simulink model "DroneModelv7"  (R2023b)
settings: Solver=VariableStepAuto  StartTime=10  StopTime=100  FixedStep=0.00001  RelTol=1e-3
undefined symbols (not defined in the file): alpha_vec_Cn0, beta_vec_Cn0, bref, Clbeta, Clda, Cm0, Cmda, Cmde, Cn0, Cnda, CX0, CXda, CXde, CYbeta, CYda, CZ0, CZda, CZde, Kalpha, Kbeta, Kp, Kphi, Kq, Kr, mass, Tc, x_cg, y_cg, z_cg
libraries: aerolibconvert2 x6, aerolibasang x3, slpidlib x3, shared6dof x1, aerolibadyn x1, aerolibatmos2 x1
settings Model: SimulationMode=accelerator  Creator=Avery  LastModifiedBy=avery
settings DataIOCC: ExternalInput=getinputstruct(op1)  InitialState=getstatestruct(op1)
settings OptimizationCC: BlockReduction=off  ConditionallyExecuteInputs=off

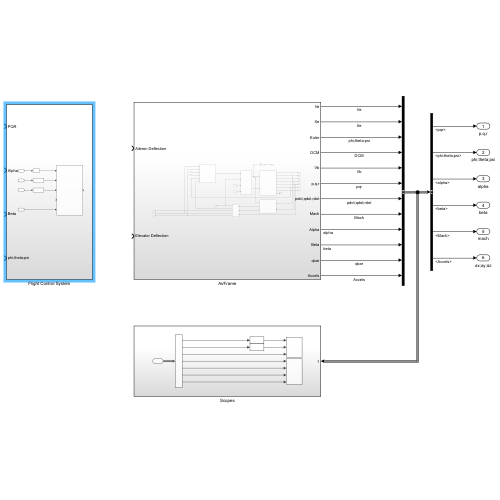
[thumbnail: Simulink's stored preview of the top-level diagram]
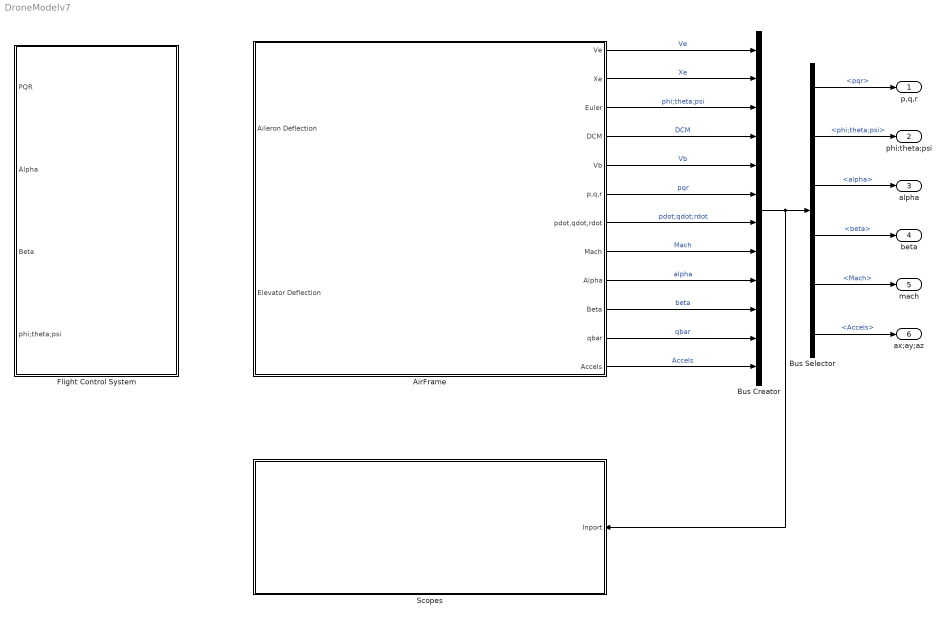
== system DroneModelv7 ==
  AirFrame : Subsystem
  Bus Creator : BusCreator  Inputs=12
  Bus Selector : BusSelector  OutputSignals=pqr,phi;theta;psi,alpha,beta,Mach,Accels
  Flight Control System : Subsystem
  Scopes : Subsystem
  p,q,r : Outport
  phi;theta;psi : Outport  Port=2
  alpha : Outport  Port=3
  beta : Outport  Port=4
  mach : Outport  Port=5
  ax;ay;az : Outport  Port=6
  wires:
  AirFrame/12(Accels) -> Bus Creator/12  "Accels"
  AirFrame/11(qbar) -> Bus Creator/11  "qbar"
  AirFrame/10(Beta) -> Bus Creator/10  "beta"
  AirFrame/9(Alpha) -> Bus Creator/9  "alpha"
  AirFrame/8(Mach) -> Bus Creator/8  "Mach"
  AirFrame/7(pdot,qdot,rdot) -> Bus Creator/7  "pdot;qdot;rdot"
  AirFrame/6(p,q,r) -> Bus Creator/6  "pqr"
  AirFrame/5(Vb) -> Bus Creator/5  "Vb"
  AirFrame/4(DCM) -> Bus Creator/4  "DCM"
  AirFrame/3(Euler) -> Bus Creator/3  "phi;theta;psi"
  AirFrame/2(Xe) -> Bus Creator/2  "Xe"
  AirFrame/1(Ve) -> Bus Creator/1  "Ve"
  Bus Selector/1 -> p,q,r/1  "<pqr>"
  Bus Selector/2 -> phi;theta;psi/1  "<phi;theta;psi>"
  Bus Selector/3 -> alpha/1  "<alpha>"
  Bus Selector/5 -> mach/1  "<Mach>"
  Bus Selector/6 -> ax;ay;az/1  "<Accels>"
  Bus Selector/4 -> beta/1  "<beta>"
  Bus Creator/1 -> Scopes/1(Inport), Bus Selector/1

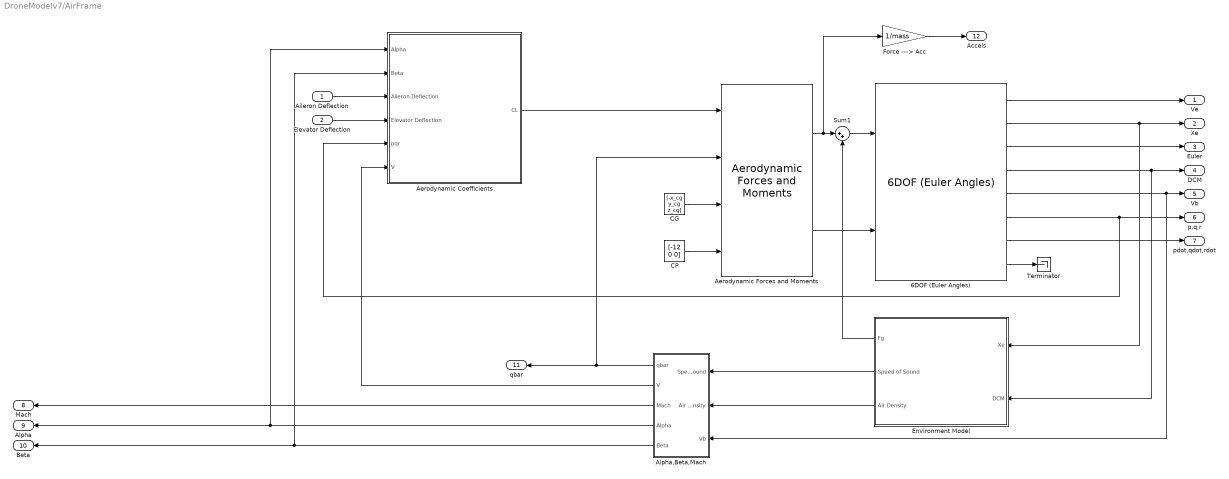
== system DroneModelv7/AirFrame ==
  Aileron Deflection : Inport  Unit=deg
  Elevator Deflection : Inport  Port=2  Unit=deg
  6DOF (Euler Angles) : shared6dof/6DOF (Euler Angles)  units=Metric (MKS)  mtype=Fixed  rep=Euler Angles  xme_0=init_pos_inertial  Vm_0=init_velo_body  eul_0=init_euler_orien  pm_0=init_body_rot  mass_0=mass  mass_e=0.5  mass_f=2.0  inertia=Inertia  inertia_e=eye(3)  inertia_f=2*eye(3)  k_quat=1.0  vre_flag=on  abi_flag=off  aMode=0  xme_statename=''  Vm_statename=''  eul_statename=''  quat_statename=''  pm_statename=''  mass_statename=''
  "Aerodynamic Forces and Moments " : aerolibadyn/Aerodynamic Forces and Moments   inputAxes=Body  outputForceAxes=Body  outputMomentAxes=Body  S=Sref  b=bref  cbar=dref
  Aerodynamic Coefficients : Subsystem
  Alpha,Beta,Mach : Subsystem
  CG : Constant  Value=[-x_cg y_cg z_cg]
  CP : Constant  Value=[-12 0 0]
  Environment Model : Subsystem
  Force ---> Acc : Gain  Gain=1/mass  SaturateOnIntegerOverflow=on  OutDataTypeStr=Inherit: Same as input  ParamDataTypeStr=Inherit: Same as input
  Sum1 : Sum  Inputs=|++  SaturateOnIntegerOverflow=on
  Terminator : Terminator
  Ve : Outport  Unit=m/s
  Xe : Outport  Port=2  Unit=meter
  Euler : Outport  Port=3  Unit=rad
  DCM : Outport  Port=4
  Vb : Outport  Port=5  Unit=m/second
  p,q,r : Outport  Port=6  Unit=rad/second
  pdot,qdot,rdot : Outport  Port=7
  Mach : Outport  Port=8
  Alpha : Outport  Port=9  Unit=rad
  Beta : Outport  Port=10  Unit=rad
  qbar : Outport  Port=11  Unit=Pa
  Accels : Outport  Port=12  Unit=m/s^2
  wires:
  6DOF (Euler Angles)/6 -> Aerodynamic Coefficients/5(pqr), p,q,r/1
  6DOF (Euler Angles)/4 -> DCM/1, Environment Model/2(DCM)
  6DOF (Euler Angles)/2 -> Xe/1, Environment Model/1(Xe)
  6DOF (Euler Angles)/5 -> Alpha,Beta,Mach/3(Vb), Vb/1
  "Aerodynamic Forces and Moments "/1 -> Force ---> Acc/1, Sum1/1
  6DOF (Euler Angles)/3 -> Euler/1
  6DOF (Euler Angles)/1 -> Ve/1
  CP/1 -> "Aerodynamic Forces and Moments "/4
  Alpha,Beta,Mach/1(qbar) -> qbar/1, "Aerodynamic Forces and Moments "/2
  CG/1 -> "Aerodynamic Forces and Moments "/3
  Alpha,Beta,Mach/4(Alpha) -> Aerodynamic Coefficients/1(Alpha), Alpha/1
  6DOF (Euler Angles)/8 -> Terminator/1
  "Aerodynamic Forces and Moments "/2 -> 6DOF (Euler Angles)/2
  6DOF (Euler Angles)/7 -> pdot,qdot,rdot/1
  Alpha,Beta,Mach/2(V) -> Aerodynamic Coefficients/6(V)
  Environment Model/1(Fg) -> Sum1/2
  Sum1/1 -> 6DOF (Euler Angles)/1
  Force ---> Acc/1 -> Accels/1
  Alpha,Beta,Mach/5(Beta) -> Aerodynamic Coefficients/2(Beta), Beta/1
  Alpha,Beta,Mach/3(Mach) -> Mach/1
  Environment Model/2(Speed of Sound) -> Alpha,Beta,Mach/1(Speed of Sound)
  Environment Model/3(Air Density) -> Alpha,Beta,Mach/2(Air Density)
  Aerodynamic Coefficients/1(CL) -> "Aerodynamic Forces and Moments "/1
  Elevator Deflection/1 -> Aerodynamic Coefficients/4(Elevator Deflection)
  Aileron Deflection/1 -> Aerodynamic Coefficients/3(Aileron Deflection)

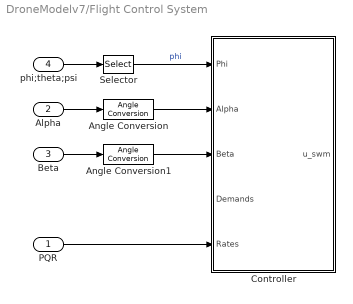
== system DroneModelv7/Flight Control System ==
  "PQR " : Inport
  Alpha : Inport  Port=2
  Beta : Inport  Port=3
  phi;theta;psi : Inport  Port=4
  Angle Conversion : aerolibconvert2/Angle Conversion  IU=rad  OU=deg
  Angle Conversion1 : aerolibconvert2/Angle Conversion  IU=rad  OU=deg
  Controller : Subsystem
  Selector : Selector  InputPortWidth=3  IndexOptions=Index vector (dialog)  Indices=[1]  OutputSizes=1
  wires:
  "PQR "/1 -> Controller/5(Rates)
  Alpha/1 -> Angle Conversion/1
  Beta/1 -> Angle Conversion1/1
  Angle Conversion1/1 -> Controller/3(Beta)
  Angle Conversion/1 -> Controller/2(Alpha)
  phi;theta;psi/1 -> Selector/1
  Selector/1 -> Controller/1(Phi)  "phi"

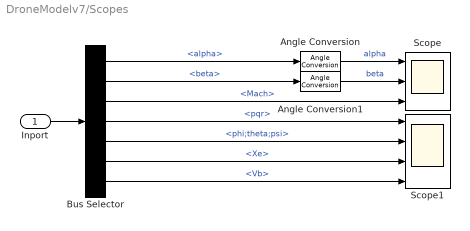
== system DroneModelv7/Scopes ==
  Inport : Inport
  Angle Conversion : aerolibconvert2/Angle Conversion  IU=rad  OU=deg
  Angle Conversion1 : aerolibconvert2/Angle Conversion  IU=rad  OU=deg
  Bus Selector : BusSelector  OutputSignals=alpha,beta,Mach,pqr,phi;theta;psi,Xe,Vb
  Scope : Scope  NumInputPorts=3
  Scope1 : Scope  NumInputPorts=4
  wires:
  Bus Selector/1 -> Angle Conversion/1  "<alpha>"
  Bus Selector/2 -> Angle Conversion1/1  "<beta>"
  Bus Selector/3 -> Scope/3  "<Mach>"
  Bus Selector/4 -> Scope1/1  "<pqr>"
  Bus Selector/5 -> Scope1/2  "<phi;theta;psi>"
  Bus Selector/6 -> Scope1/3  "<Xe>"
  Inport/1 -> Bus Selector/1
  Angle Conversion1/1 -> Scope/2  "beta"
  Angle Conversion/1 -> Scope/1  "alpha"
  Bus Selector/7 -> Scope1/4  "<Vb>"

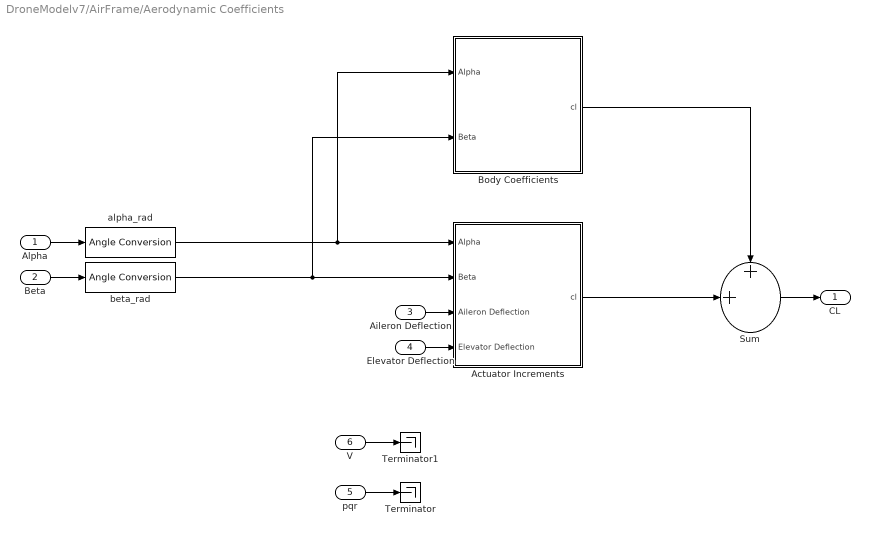
== system DroneModelv7/AirFrame/Aerodynamic Coefficients ==
  Alpha : Inport
  Beta : Inport  Port=2
  Aileron Deflection : Inport  Port=3
  Elevator Deflection : Inport  Port=4
  pqr : Inport  Port=5
  V : Inport  Port=6
  Actuator Increments : Subsystem
  Body Coefficients : Subsystem
  Sum : Sum  Inputs=++|  InputSameDT=on  SaturateOnIntegerOverflow=on  OutDataTypeStr=Inherit: Same as first input
  Terminator : Terminator
  Terminator1 : Terminator
  alpha_rad : aerolibconvert2/Angle Conversion  IU=rad  OU=deg
  beta_rad : aerolibconvert2/Angle Conversion  IU=rad  OU=deg
  CL : Outport
  wires:
  Elevator Deflection/1 -> Actuator Increments/4(Elevator Deflection)
  Beta/1 -> beta_rad/1
  Alpha/1 -> alpha_rad/1
  Body Coefficients/1(cl) -> Sum/1
  Aileron Deflection/1 -> Actuator Increments/3(Aileron Deflection)
  Actuator Increments/1(cl) -> Sum/2
  Sum/1 -> CL/1
  alpha_rad/1 -> Body Coefficients/1(Alpha), Actuator Increments/1(Alpha)
  beta_rad/1 -> Body Coefficients/2(Beta), Actuator Increments/2(Beta)
  pqr/1 -> Terminator/1
  V/1 -> Terminator1/1

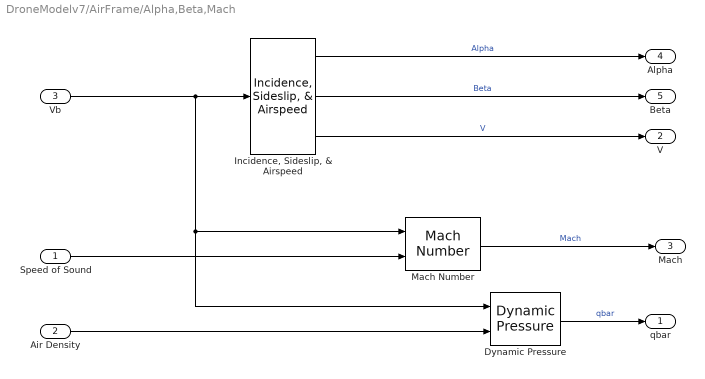
== system DroneModelv7/AirFrame/Alpha,Beta,Mach ==
  Speed of Sound : Inport
  Air Density : Inport  Port=2
  Vb : Inport  Port=3  PortDimensions=3
  Dynamic Pressure : aerolibasang/Dynamic Pressure
  "Incidence, Sideslip, & Airspeed" : aerolibasang/Incidence, Sideslip, & Airspeed
  Mach Number : aerolibasang/Mach Number
  qbar : Outport  Unit=Pa  InitialOutput=0  VectorParamsAs1DForOutWhenUnconnected=off
  V : Outport  Port=2  Unit=m/s  VectorParamsAs1DForOutWhenUnconnected=off
  Mach : Outport  Port=3  VectorParamsAs1DForOutWhenUnconnected=off
  Alpha : Outport  Port=4  Unit=rad  VectorParamsAs1DForOutWhenUnconnected=off
  Beta : Outport  Port=5  Unit=rad  VectorParamsAs1DForOutWhenUnconnected=off
  wires:
  Air Density/1 -> Dynamic Pressure/2
  "Incidence, Sideslip, & Airspeed"/2 -> Beta/1  "Beta"
  "Incidence, Sideslip, & Airspeed"/1 -> Alpha/1  "Alpha"
  Vb/1 -> Dynamic Pressure/1, Mach Number/1, "Incidence, Sideslip, & Airspeed"/1
  Mach Number/1 -> Mach/1  "Mach"
  Dynamic Pressure/1 -> qbar/1  "qbar"
  Speed of Sound/1 -> Mach Number/2
  "Incidence, Sideslip, & Airspeed"/3 -> V/1  "V"

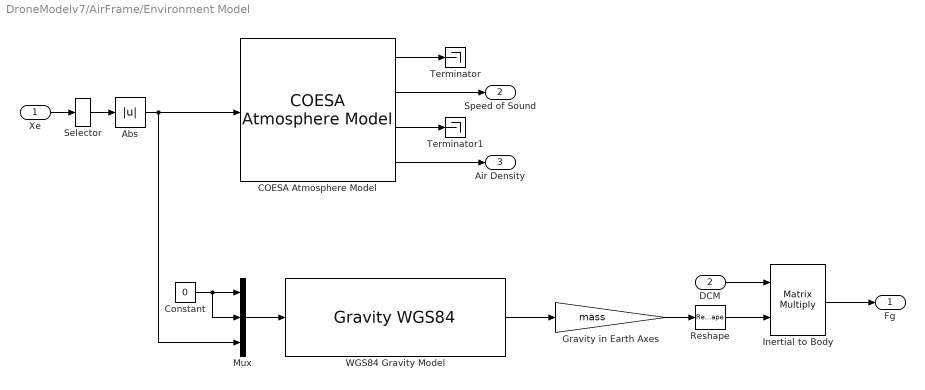
== system DroneModelv7/AirFrame/Environment Model ==
  Xe : Inport  Unit=meter  PortDimensions=3
  DCM : Inport  Port=2
  Abs : Abs  SaturateOnIntegerOverflow=off
  COESA Atmosphere Model : aerolibatmos2/COESA Atmosphere Model  units=Metric (MKS)  spec=1976 COESA-extended U.S. Standard Atmosphere  model=Profile  profile_var=High temperature  profile_percent=1%  profile_alt=5 km (16404 ft)  envelope_var=High temperature  envelope_percent=1%  action=Warning
  Constant : Constant  Value=0
  Gravity in Earth Axes : Gain  Gain=mass  SaturateOnIntegerOverflow=on  ParamDataTypeStr=Inherit: Same as input
  Inertial to Body : Product  Multiplication=Matrix(*)  InputSameDT=on  SaturateOnIntegerOverflow=on  OutDataTypeStr=Inherit: Same as first input
  Mux : Mux  Inputs=3
  Reshape : Reshape
  Selector : Selector  InputPortWidth=3  IndexOptions=Index vector (dialog)  Indices=[3]  OutputSizes=1
  Terminator : Terminator
  Terminator1 : Terminator
  "WGS84 Gravity Model  " : GravityWGS84  action=None
  Fg : Outport
  Speed of Sound : Outport  Port=2
  Air Density : Outport  Port=3
  wires:
  COESA Atmosphere Model/1 -> Terminator/1
  COESA Atmosphere Model/3 -> Terminator1/1
  COESA Atmosphere Model/2 -> Speed of Sound/1
  COESA Atmosphere Model/4 -> Air Density/1
  Reshape/1 -> Inertial to Body/2
  Gravity in Earth Axes/1 -> Reshape/1
  DCM/1 -> Inertial to Body/1
  Inertial to Body/1 -> Fg/1
  Abs/1 -> Mux/3, COESA Atmosphere Model/1
  Constant/1 -> Mux/1, Mux/2
  Mux/1 -> "WGS84 Gravity Model  "/1
  "WGS84 Gravity Model  "/1 -> Gravity in Earth Axes/1
  Xe/1 -> Selector/1
  Selector/1 -> Abs/1

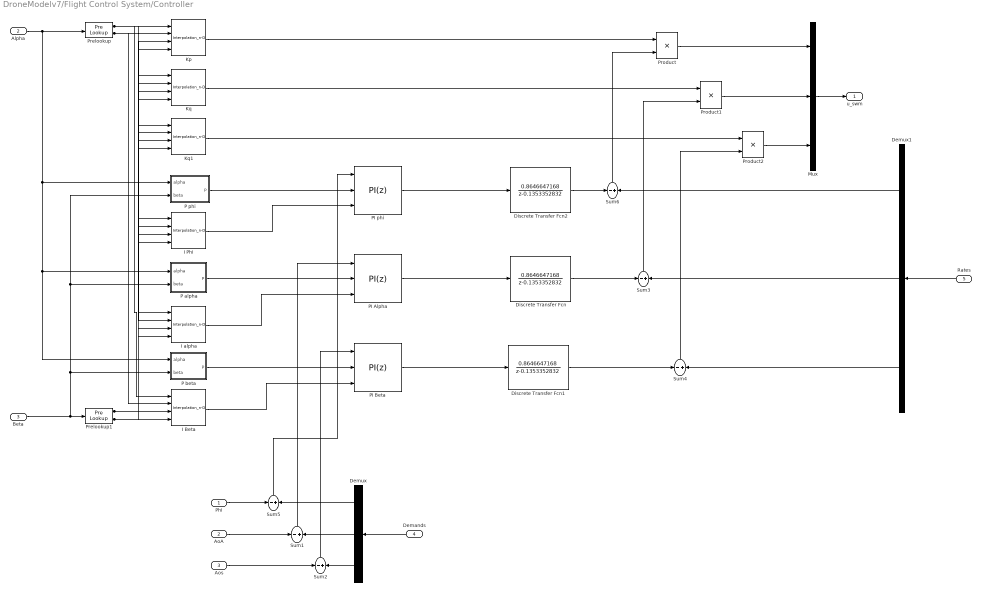
== system DroneModelv7/Flight Control System/Controller ==
  Phi : Inport
  Alpha : Inport  Port=2
  Beta : Inport  Port=3
  Demands : Inport  Port=4
  Rates : Inport  Port=5
  AoA : InportShadow  Port=2
  Aos : InportShadow  Port=3
  Demux : Demux  Outputs=3
  Demux1 : Demux  Outputs=3
  Discrete Transfer Fcn : DiscreteTransferFcn  Numerator=0.8646647168  Denominator=[1, -0.1353352832]  SampleTime=Tc  SaturateOnIntegerOverflow=on
  Discrete Transfer Fcn1 : DiscreteTransferFcn  Numerator=0.8646647168  Denominator=[1, -0.1353352832]  SampleTime=Tc  SaturateOnIntegerOverflow=on
  Discrete Transfer Fcn2 : DiscreteTransferFcn  Numerator=0.8646647168  Denominator=[1, -0.1353352832]  SampleTime=Tc  SaturateOnIntegerOverflow=on
  I Beta : Interpolation_n-D  Table=Kbeta  RemoveProtectionIndex=on
  I Phi : Interpolation_n-D  Table=Kphi  RemoveProtectionIndex=on
  I alpha : Interpolation_n-D  Table=Kalpha  RemoveProtectionIndex=on
  Kp : Interpolation_n-D  Table=Kp  RemoveProtectionIndex=on
  Kq : Interpolation_n-D  Table=Kq  RemoveProtectionIndex=on
  Kq1 : Interpolation_n-D  Table=Kr  RemoveProtectionIndex=on
  Mux : Mux  Inputs=3
  P alpha : MATLAB Function  TreatAsAtomicUnit=on
  P beta : MATLAB Function  TreatAsAtomicUnit=on
  P phi : MATLAB Function  TreatAsAtomicUnit=on
  PI Alpha : slpidlib/PID Controller  Controller=PI  Form=Parallel  TimeDomain=Discrete-time  UseExternalTs=off  SampleTime=Tc  IntegratorMethod=Forward Euler  FilterMethod=Forward Euler  ControllerParametersSource=external  P=1  I=1  UseKiTs=off  D=0  N=100  UseFilter=on  TunerSelectOption=Transfer Function Based (PID Tuner App)  InitialConditionSource=internal  InitialConditionForIntegrator=0  InitialConditionForFilter=0  DifferentiatorICPrevScaledInput=0  ExternalReset=none  TrackingMode=off  Kt=1  LimitOutput=off  SatLimitsSource=internal  UpperSaturationLimit=inf  LowerSaturationLimit=-inf  LinearizeAsGain=on  AntiWindupMode=none  Kb=1  LimitIntegrator=off  UpperIntegratorSaturationLimit=inf  LowerIntegratorSaturationLimit=-inf  POutMin=[]  POutMax=[]  IOutMin=[]  IOutMax=[]  DOutMin=[]  DOutMax=[]  NOutMin=[]  NOutMax=[]  SumOutMin=[]  SumOutMax=[]  SaturationOutMin=[]  SaturationOutMax=[]  PParamMin=[]  PParamMax=[]  IParamMin=[]  IParamMax=[]  DParamMin=[]  DParamMax=[]  NParamMin=[]  NParamMax=[]  KbParamMin=[]  KbParamMax=[]  KtParamMin=[]  KtParamMax=[]  KbOutMin=[]  KbOutMax=[]  KtOutMin=[]  KtOutMax=[]  IntegratorOutMin=[]  IntegratorOutMax=[]  FilterOutMin=[]  FilterOutMax=[]  SumI1OutMin=[]  SumI1OutMax=[]  SumI2OutMin=[]  SumI2OutMax=[]  SumI3OutMin=[]  SumI3OutMax=[]  SumI4OutMin=[]  SumI4OutMax=[]  SumDOutMin=[]  SumDOutMax=[]  DifferentiatorOutMin=[]  DifferentiatorOutMax=[]  FilterDiffOutCoefMin=[]  FilterDiffOutCoefMax=[]  ReciprocalOutMin=[]  ReciprocalOutMax=[]  SumDenOutMin=[]  SumDenOutMax=[]  SumNumOutMin=[]  SumNumOutMax=[]  DivideOutMin=[]  DivideOutMax=[]  UdiffTsProdOutMin=[]  UdiffTsProdOutMax=[]  NTsProdOutMin=[]  NTsProdOutMax=[]  UintegralTsProdOutMin=[]  UintegralTsProdOutMax=[]  UngainTsProdOutMin=[]  UngainTsProdOutMax=[]  ClampingZeroOutDataTypeStr=Inherit: Inherit via back propagation  ClampingZeroOutMin=[]  ClampingZeroOutMax=[]  FilterDenConstantOutDataTypeStr=Inherit: Inherit via back propagation  FilterDenConstantOutMin=[]  FilterDenConstantOutMax=[]  PCopyOutDataTypeStr=Inherit: Inherit via back propagation  PCopyOutMin=[]  PCopyOutMax=[]  NCopyOutDataTypeStr=Inherit: Inherit via back propagation  NCopyOutMin=[]  NCopyOutMax=[]  IntegratorContinuousStateAttributes=''  IntegratorStateMustResolveToSignalObject=off  IntegratorRTWStateStorageClass=Auto  FilterContinuousStateAttributes=''  FilterStateMustResolveToSignalObject=off  FilterRTWStateStorageClass=Auto  ParallelPVariant=ExternalParameters  IdealPVariant=Disabled  IVariant=ExternalParameters  DVariant=Disabled  IntegratorVariant=Discrete  SatVariant=Disabled  AWVariant=Passthrough  PCopyVariant=Disabled  TRVariant=Disabled  FdbkBlocksVariant=Forward  IdealPFdbkVariant=Disabled  SatFdbkVariant=Disabled  DerivativeFilterVariant=Disabled  NVariant=Disabled  NCopyVariant=Disabled_SignalSpec  FilterICVariant=Disabled  IntegratorICVariant=InternalICs  ExternalResetVariant=Disabled  TRSumVariant=Passthrough  SumFdbkVariant=Disabled  SumVariant=Sum_PI  TsampFilterVariant=InternalTs  TsampNgainVariant=Passthrough  TsampIntegralVariant=Disabled_SignalSpec  ExternalSaturationOutDataTypeStr=Inherit: Same as second input
  PI Beta : slpidlib/PID Controller  Controller=PI  Form=Parallel  TimeDomain=Discrete-time  UseExternalTs=off  SampleTime=Tc  IntegratorMethod=Forward Euler  FilterMethod=Forward Euler  ControllerParametersSource=external  P=1  I=1  UseKiTs=off  D=0  N=100  UseFilter=on  TunerSelectOption=Transfer Function Based (PID Tuner App)  InitialConditionSource=internal  InitialConditionForIntegrator=0  InitialConditionForFilter=0  DifferentiatorICPrevScaledInput=0  ExternalReset=none  TrackingMode=off  Kt=1  LimitOutput=off  SatLimitsSource=internal  UpperSaturationLimit=inf  LowerSaturationLimit=-inf  LinearizeAsGain=on  AntiWindupMode=none  Kb=1  LimitIntegrator=off  UpperIntegratorSaturationLimit=inf  LowerIntegratorSaturationLimit=-inf  POutMin=[]  POutMax=[]  IOutMin=[]  IOutMax=[]  DOutMin=[]  DOutMax=[]  NOutMin=[]  NOutMax=[]  SumOutMin=[]  SumOutMax=[]  SaturationOutMin=[]  SaturationOutMax=[]  PParamMin=[]  PParamMax=[]  IParamMin=[]  IParamMax=[]  DParamMin=[]  DParamMax=[]  NParamMin=[]  NParamMax=[]  KbParamMin=[]  KbParamMax=[]  KtParamMin=[]  KtParamMax=[]  KbOutMin=[]  KbOutMax=[]  KtOutMin=[]  KtOutMax=[]  IntegratorOutMin=[]  IntegratorOutMax=[]  FilterOutMin=[]  FilterOutMax=[]  SumI1OutMin=[]  SumI1OutMax=[]  SumI2OutMin=[]  SumI2OutMax=[]  SumI3OutMin=[]  SumI3OutMax=[]  SumI4OutMin=[]  SumI4OutMax=[]  SumDOutMin=[]  SumDOutMax=[]  DifferentiatorOutMin=[]  DifferentiatorOutMax=[]  FilterDiffOutCoefMin=[]  FilterDiffOutCoefMax=[]  ReciprocalOutMin=[]  ReciprocalOutMax=[]  SumDenOutMin=[]  SumDenOutMax=[]  SumNumOutMin=[]  SumNumOutMax=[]  DivideOutMin=[]  DivideOutMax=[]  UdiffTsProdOutMin=[]  UdiffTsProdOutMax=[]  NTsProdOutMin=[]  NTsProdOutMax=[]  UintegralTsProdOutMin=[]  UintegralTsProdOutMax=[]  UngainTsProdOutMin=[]  UngainTsProdOutMax=[]  ClampingZeroOutDataTypeStr=Inherit: Inherit via back propagation  ClampingZeroOutMin=[]  ClampingZeroOutMax=[]  FilterDenConstantOutDataTypeStr=Inherit: Inherit via back propagation  FilterDenConstantOutMin=[]  FilterDenConstantOutMax=[]  PCopyOutDataTypeStr=Inherit: Inherit via back propagation  PCopyOutMin=[]  PCopyOutMax=[]  NCopyOutDataTypeStr=Inherit: Inherit via back propagation  NCopyOutMin=[]  NCopyOutMax=[]  IntegratorContinuousStateAttributes=''  IntegratorStateMustResolveToSignalObject=off  IntegratorRTWStateStorageClass=Auto  FilterContinuousStateAttributes=''  FilterStateMustResolveToSignalObject=off  FilterRTWStateStorageClass=Auto  ParallelPVariant=ExternalParameters  IdealPVariant=Disabled  IVariant=ExternalParameters  DVariant=Disabled  IntegratorVariant=Discrete  SatVariant=Disabled  AWVariant=Passthrough  PCopyVariant=Disabled  TRVariant=Disabled  FdbkBlocksVariant=Forward  IdealPFdbkVariant=Disabled  SatFdbkVariant=Disabled  DerivativeFilterVariant=Disabled  NVariant=Disabled  NCopyVariant=Disabled_SignalSpec  FilterICVariant=Disabled  IntegratorICVariant=InternalICs  ExternalResetVariant=Disabled  TRSumVariant=Passthrough  SumFdbkVariant=Disabled  SumVariant=Sum_PI  TsampFilterVariant=InternalTs  TsampNgainVariant=Passthrough  TsampIntegralVariant=Disabled_SignalSpec  ExternalSaturationOutDataTypeStr=Inherit: Same as second input
  PI phi : slpidlib/PID Controller  Controller=PI  Form=Parallel  TimeDomain=Discrete-time  UseExternalTs=off  SampleTime=Tc  IntegratorMethod=Forward Euler  FilterMethod=Forward Euler  ControllerParametersSource=external  P=1  I=1  UseKiTs=off  D=0  N=100  UseFilter=on  TunerSelectOption=Transfer Function Based (PID Tuner App)  InitialConditionSource=internal  InitialConditionForIntegrator=0  InitialConditionForFilter=0  DifferentiatorICPrevScaledInput=0  ExternalReset=none  TrackingMode=off  Kt=1  LimitOutput=off  SatLimitsSource=internal  UpperSaturationLimit=inf  LowerSaturationLimit=-inf  LinearizeAsGain=on  AntiWindupMode=none  Kb=1  LimitIntegrator=off  UpperIntegratorSaturationLimit=inf  LowerIntegratorSaturationLimit=-inf  POutMin=[]  POutMax=[]  IOutMin=[]  IOutMax=[]  DOutMin=[]  DOutMax=[]  NOutMin=[]  NOutMax=[]  SumOutMin=[]  SumOutMax=[]  SaturationOutMin=[]  SaturationOutMax=[]  PParamMin=[]  PParamMax=[]  IParamMin=[]  IParamMax=[]  DParamMin=[]  DParamMax=[]  NParamMin=[]  NParamMax=[]  KbParamMin=[]  KbParamMax=[]  KtParamMin=[]  KtParamMax=[]  KbOutMin=[]  KbOutMax=[]  KtOutMin=[]  KtOutMax=[]  IntegratorOutMin=[]  IntegratorOutMax=[]  FilterOutMin=[]  FilterOutMax=[]  SumI1OutMin=[]  SumI1OutMax=[]  SumI2OutMin=[]  SumI2OutMax=[]  SumI3OutMin=[]  SumI3OutMax=[]  SumI4OutMin=[]  SumI4OutMax=[]  SumDOutMin=[]  SumDOutMax=[]  DifferentiatorOutMin=[]  DifferentiatorOutMax=[]  FilterDiffOutCoefMin=[]  FilterDiffOutCoefMax=[]  ReciprocalOutMin=[]  ReciprocalOutMax=[]  SumDenOutMin=[]  SumDenOutMax=[]  SumNumOutMin=[]  SumNumOutMax=[]  DivideOutMin=[]  DivideOutMax=[]  UdiffTsProdOutMin=[]  UdiffTsProdOutMax=[]  NTsProdOutMin=[]  NTsProdOutMax=[]  UintegralTsProdOutMin=[]  UintegralTsProdOutMax=[]  UngainTsProdOutMin=[]  UngainTsProdOutMax=[]  ClampingZeroOutDataTypeStr=Inherit: Inherit via back propagation  ClampingZeroOutMin=[]  ClampingZeroOutMax=[]  FilterDenConstantOutDataTypeStr=Inherit: Inherit via back propagation  FilterDenConstantOutMin=[]  FilterDenConstantOutMax=[]  PCopyOutDataTypeStr=Inherit: Inherit via back propagation  PCopyOutMin=[]  PCopyOutMax=[]  NCopyOutDataTypeStr=Inherit: Inherit via back propagation  NCopyOutMin=[]  NCopyOutMax=[]  IntegratorContinuousStateAttributes=''  IntegratorStateMustResolveToSignalObject=off  IntegratorRTWStateStorageClass=Auto  FilterContinuousStateAttributes=''  FilterStateMustResolveToSignalObject=off  FilterRTWStateStorageClass=Auto  ParallelPVariant=ExternalParameters  IdealPVariant=Disabled  IVariant=ExternalParameters  DVariant=Disabled  IntegratorVariant=Discrete  SatVariant=Disabled  AWVariant=Passthrough  PCopyVariant=Disabled  TRVariant=Disabled  FdbkBlocksVariant=Forward  IdealPFdbkVariant=Disabled  SatFdbkVariant=Disabled  DerivativeFilterVariant=Disabled  NVariant=Disabled  NCopyVariant=Disabled_SignalSpec  FilterICVariant=Disabled  IntegratorICVariant=InternalICs  ExternalResetVariant=Disabled  TRSumVariant=Passthrough  SumFdbkVariant=Disabled  SumVariant=Sum_PI  TsampFilterVariant=InternalTs  TsampNgainVariant=Passthrough  TsampIntegralVariant=Disabled_SignalSpec  ExternalSaturationOutDataTypeStr=Inherit: Same as second input
  Prelookup : PreLookup  BreakpointsData=a_vec  BeginIndexSearchUsingPreviousIndexResult=on  ExtrapMethod=Linear
  Prelookup1 : PreLookup  BreakpointsData=b_vec  BeginIndexSearchUsingPreviousIndexResult=on  ExtrapMethod=Linear
  Product : Product
  Product1 : Product
  Product2 : Product
  Sum{1..6} (6 alike) : Sum  Inputs=-|+
  u_swm : Outport
  wires:
  Alpha/1 -> P phi/1(alpha), P beta/1(alpha), P alpha/1(alpha), Prelookup/1
  Prelookup/1 -> I Phi/1, I alpha/1, Kp/1, I Beta/1, Kq/1, Kq1/1
  Prelookup/2 -> I Phi/2, I alpha/2, Kp/2, I Beta/2, Kq/2, Kq1/2
  Beta/1 -> P phi/2(beta), P alpha/2(beta), P beta/2(beta), Prelookup1/1
  Prelookup1/1 -> I Beta/3, I Phi/3, I alpha/3, Kp/3, Kq/3, Kq1/3
  Prelookup1/2 -> I Phi/4, I alpha/4, Kp/4, I Beta/4, Kq/4, Kq1/4
  Aos/1 -> Sum2/1
  AoA/1 -> Sum1/1
  Demands/1 -> Demux/1
  Sum1/1 -> PI Alpha/1
  Sum2/1 -> PI Beta/1
  P beta/1(P) -> PI Beta/2
  I Beta/1 -> PI Beta/3
  P alpha/1(P) -> PI Alpha/2
  I alpha/1 -> PI Alpha/3
  PI Alpha/1 -> Discrete Transfer Fcn/1
  Discrete Transfer Fcn/1 -> Sum3/1
  Discrete Transfer Fcn1/1 -> Sum4/1
  P phi/1(P) -> PI phi/2
  I Phi/1 -> PI phi/3
  Demux/3 -> Sum2/2
  Demux/2 -> Sum1/2
  Phi/1 -> Sum5/1
  Demux/1 -> Sum5/2
  Sum5/1 -> PI phi/1
  PI phi/1 -> Discrete Transfer Fcn2/1
  Discrete Transfer Fcn2/1 -> Sum6/1
  Kp/1 -> Product/1
  Kq/1 -> Product1/1
  Kq1/1 -> Product2/1
  Sum6/1 -> Product/2
  Sum3/1 -> Product1/2
  Sum4/1 -> Product2/2
  PI Beta/1 -> Discrete Transfer Fcn1/1
  Product/1 -> Mux/1
  Product1/1 -> Mux/2
  Product2/1 -> Mux/3
  Mux/1 -> u_swm/1
  Demux1/1 -> Sum6/2
  Demux1/2 -> Sum3/2
  Demux1/3 -> Sum4/2
  Rates/1 -> Demux1/1

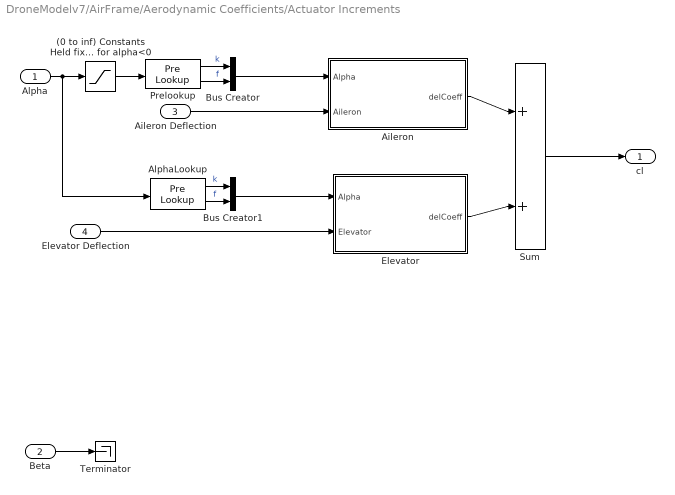
== system DroneModelv7/AirFrame/Aerodynamic Coefficients/Actuator Increments ==
  Alpha : Inport
  Beta : Inport  Port=2
  Aileron Deflection : Inport  Port=3
  Elevator Deflection : Inport  Port=4
  (0 to inf) Constants Held fixed for alpha<0 : Saturate  UpperLimit=inf  LowerLimit=0
  Aileron : Subsystem  AncestorBlock=|
      | aeroblk_lib_HL20/HL20
      | Airframe/Aerodynamic
      | Coefficients/Actuator
      | Increments/Aileron
  AlphaLookup : PreLookup  BreakpointsData=alpha_vec_0  BeginIndexSearchUsingPreviousIndexResult=on  ExtrapMethod=Linear
  Bus Creator : BusCreator  Inputs=2
  Bus Creator1 : BusCreator  Inputs=2
  Elevator : Subsystem  AncestorBlock=|
      | aeroblk_lib_HL20/HL20
      | Airframe/Aerodynamic
      | Coefficients/Actuator
      | Increments/Elevator
  Prelookup : PreLookup  BreakpointsData=alpha_vec_0  BeginIndexSearchUsingPreviousIndexResult=on  ExtrapMethod=Linear
  Sum : Sum  Inputs=+|+  InputSameDT=on  SaturateOnIntegerOverflow=on
  Terminator : Terminator
  cl : Outport
  wires:
  Beta/1 -> Terminator/1
  Alpha/1 -> AlphaLookup/1, (0 to inf) Constants Held fixed for alpha<0/1
  (0 to inf) Constants Held fixed for alpha<0/1 -> Prelookup/1
  Prelookup/1 -> Bus Creator/1  "k"
  Prelookup/2 -> Bus Creator/2  "f"
  Bus Creator/1 -> Aileron/1(Alpha)
  AlphaLookup/1 -> Bus Creator1/1  "k"
  AlphaLookup/2 -> Bus Creator1/2  "f"
  Bus Creator1/1 -> Elevator/1(Alpha)
  Elevator/1(delCoeff) -> Sum/2
  Aileron/1(delCoeff) -> Sum/1
  Sum/1 -> cl/1
  Elevator Deflection/1 -> Elevator/2(Elevator)
  Aileron Deflection/1 -> Aileron/2(Aileron)

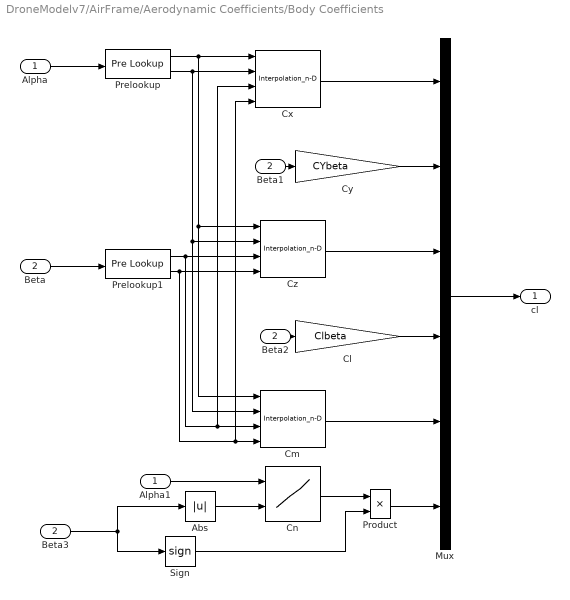
== system DroneModelv7/AirFrame/Aerodynamic Coefficients/Body Coefficients ==
  Alpha : Inport
  Beta : Inport  Port=2
  " Cn" : Lookup_n-D  BreakpointsForDimension1=alpha_vec_Cn0  BreakpointsForDimension2=beta_vec_Cn0  Table=Cn0  InternalRulePriority=Speed  RndMeth=Simplest
      settings: InputPortMap=u0,u1
  Abs : Abs
  Alpha1 : InportShadow
  Beta1 : InportShadow  Port=2
  Beta2 : InportShadow  Port=2
  Beta3 : InportShadow  Port=2
  Cl : Gain  Gain=Clbeta  SaturateOnIntegerOverflow=on  OutDataTypeStr=Inherit: Same as input  ParamDataTypeStr=Inherit: Same as input
  Cm : Interpolation_n-D  Table=Cm0'  RemoveProtectionIndex=on  SaturateOnIntegerOverflow=on
  Cx : Interpolation_n-D  Table=CX0'  RemoveProtectionIndex=on  SaturateOnIntegerOverflow=on
  Cy : Gain  Gain=CYbeta  SaturateOnIntegerOverflow=on  OutDataTypeStr=Inherit: Same as input  ParamDataTypeStr=Inherit: Same as input
  Cz : Interpolation_n-D  Table=CZ0'  RemoveProtectionIndex=on  SaturateOnIntegerOverflow=on
  Mux : Mux  Inputs=6
  Prelookup : PreLookup  BreakpointsData=alpha_vec_0  BeginIndexSearchUsingPreviousIndexResult=on  ExtrapMethod=Linear
  Prelookup1 : PreLookup  BreakpointsData=beta_vec_0  BeginIndexSearchUsingPreviousIndexResult=on  ExtrapMethod=Linear
  Product : Product  InputSameDT=on  SaturateOnIntegerOverflow=on  OutDataTypeStr=Inherit: Same as first input
  Sign : Signum
  cl : Outport
  wires:
  Alpha/1 -> Prelookup/1
  Prelookup/1 -> Cx/1, Cm/1, Cz/1
  Prelookup/2 -> Cx/2, Cm/2, Cz/2
  Prelookup1/1 -> Cx/3, Cm/3, Cz/3
  Prelookup1/2 -> Cx/4, Cm/4, Cz/4
  Beta/1 -> Prelookup1/1
  Beta1/1 -> Cy/1
  Beta2/1 -> Cl/1
  Alpha1/1 -> " Cn"/1
  Cz/1 -> Mux/3
  Cy/1 -> Mux/2
  Cx/1 -> Mux/1
  Cl/1 -> Mux/4
  Cm/1 -> Mux/5
  Product/1 -> Mux/6
  Beta3/1 -> Sign/1, Abs/1
  Abs/1 -> " Cn"/2
  Sign/1 -> Product/2
  " Cn"/1 -> Product/1
  Mux/1 -> cl/1

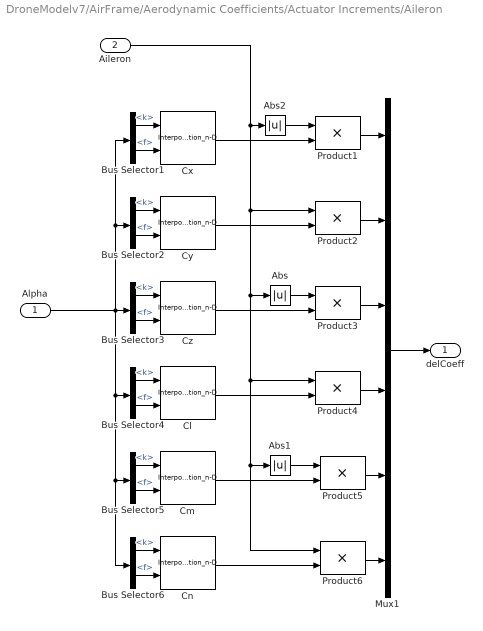
== system DroneModelv7/AirFrame/Aerodynamic Coefficients/Actuator Increments/Aileron ==
  Alpha : Inport
  Aileron : Inport  Port=2
  Abs : Abs
  Abs1 : Abs
  Abs2 : Abs
  Bus Selector{1..6} (6 alike) : BusSelector  OutputSignals=k,f
  Cl : Interpolation_n-D  NumberOfTableDimensions=1  Table=Clda  RemoveProtectionIndex=on  SaturateOnIntegerOverflow=on
      settings: InputPortMap=u0,u1
  Cm : Interpolation_n-D  NumberOfTableDimensions=1  Table=Cmda  RemoveProtectionIndex=on  SaturateOnIntegerOverflow=on
      settings: InputPortMap=u0,u1
  Cn : Interpolation_n-D  NumberOfTableDimensions=1  Table=Cnda  RemoveProtectionIndex=on  SaturateOnIntegerOverflow=on
      settings: InputPortMap=u0,u1
  Cx : Interpolation_n-D  NumberOfTableDimensions=1  Table=CXda  RemoveProtectionIndex=on  SaturateOnIntegerOverflow=on
      settings: InputPortMap=u0,u1
  Cy : Interpolation_n-D  NumberOfTableDimensions=1  Table=CYda  RemoveProtectionIndex=on  SaturateOnIntegerOverflow=on
      settings: InputPortMap=u0,u1
  Cz : Interpolation_n-D  NumberOfTableDimensions=1  Table=CZda  RemoveProtectionIndex=on  SaturateOnIntegerOverflow=on
      settings: InputPortMap=u0,u1
  Mux1 : Mux  Inputs=6
  Product{1..6} (6 alike) : Product  InputSameDT=on  SaturateOnIntegerOverflow=on  OutDataTypeStr=Inherit: Same as first input
  delCoeff : Outport  VectorParamsAs1DForOutWhenUnconnected=off
  wires:
  Bus Selector6/2 -> Cn/2  "<f>"
  Bus Selector6/1 -> Cn/1  "<k>"
  Bus Selector5/2 -> Cm/2  "<f>"
  Bus Selector5/1 -> Cm/1  "<k>"
  Bus Selector4/2 -> Cl/2  "<f>"
  Bus Selector4/1 -> Cl/1  "<k>"
  Bus Selector3/2 -> Cz/2  "<f>"
  Bus Selector3/1 -> Cz/1  "<k>"
  Bus Selector2/2 -> Cy/2  "<f>"
  Bus Selector2/1 -> Cy/1  "<k>"
  Bus Selector1/2 -> Cx/2  "<f>"
  Bus Selector1/1 -> Cx/1  "<k>"
  Alpha/1 -> Bus Selector3/1, Bus Selector4/1, Bus Selector6/1, Bus Selector5/1, Bus Selector2/1, Bus Selector1/1
  Abs2/1 -> Product1/1
  Abs1/1 -> Product5/1
  Abs/1 -> Product3/1
  Aileron/1 -> Abs2/1, Product2/1, Abs/1, Product4/1, Abs1/1, Product6/1
  Product6/1 -> Mux1/6
  Cn/1 -> Product6/2
  Product5/1 -> Mux1/5
  Cm/1 -> Product5/2
  Product4/1 -> Mux1/4
  Cl/1 -> Product4/2
  Cz/1 -> Product3/2
  Product3/1 -> Mux1/3
  Cy/1 -> Product2/2
  Product2/1 -> Mux1/2
  Cx/1 -> Product1/2
  Product1/1 -> Mux1/1
  Mux1/1 -> delCoeff/1

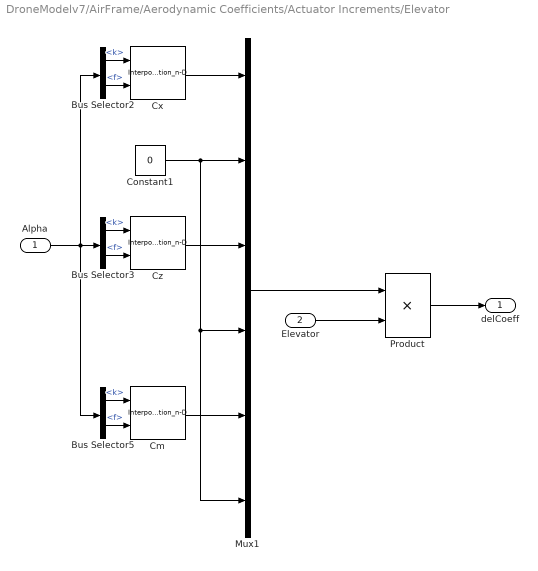
== system DroneModelv7/AirFrame/Aerodynamic Coefficients/Actuator Increments/Elevator ==
  Alpha : Inport
  Elevator : Inport  Port=2
  Bus Selector2 : BusSelector  OutputSignals=k,f
  Bus Selector3 : BusSelector  OutputSignals=k,f
  Bus Selector5 : BusSelector  OutputSignals=k,f
  Cm : Interpolation_n-D  NumberOfTableDimensions=1  Table=Cmde  RemoveProtectionIndex=on  SaturateOnIntegerOverflow=on
      settings: InputPortMap=u0,u1
  Constant1 : Constant  Value=0
  Cx : Interpolation_n-D  NumberOfTableDimensions=1  Table=CXde  RemoveProtectionIndex=on  SaturateOnIntegerOverflow=on
      settings: InputPortMap=u0,u1
  Cz : Interpolation_n-D  NumberOfTableDimensions=1  Table=CZde  RemoveProtectionIndex=on  SaturateOnIntegerOverflow=on
      settings: InputPortMap=u0,u1
  Mux1 : Mux  Inputs=6
  Product : Product  InputSameDT=on  SaturateOnIntegerOverflow=on  OutDataTypeStr=Inherit: Same as first input
  delCoeff : Outport  VectorParamsAs1DForOutWhenUnconnected=off
  wires:
  Bus Selector5/2 -> Cm/2  "<f>"
  Bus Selector5/1 -> Cm/1  "<k>"
  Bus Selector3/2 -> Cz/2  "<f>"
  Bus Selector3/1 -> Cz/1  "<k>"
  Bus Selector2/2 -> Cx/2  "<f>"
  Bus Selector2/1 -> Cx/1  "<k>"
  Constant1/1 -> Mux1/6, Mux1/4, Mux1/2
  Cm/1 -> Mux1/5
  Cz/1 -> Mux1/3
  Cx/1 -> Mux1/1
  Alpha/1 -> Bus Selector5/1, Bus Selector3/1, Bus Selector2/1
  Mux1/1 -> Product/1
  Product/1 -> delCoeff/1
  Elevator/1 -> Product/2

== matlab function DroneModelv7/Flight Control System/Controller/P alpha ==
  data: alpha input; P output; beta input
function P = fcn(alpha,beta)

P = 0.05;

== matlab function DroneModelv7/Flight Control System/Controller/P beta ==
  data: alpha input; P output; beta input
function P = fcn(alpha,beta)

P = -0.05;

== matlab function DroneModelv7/Flight Control System/Controller/P phi ==
  data: alpha input; P output; beta input
function P = fcn(alpha,beta)

P = 0.05;
